simulink model "foureightbits_thirtytwobit"  (Simulink 7.8)
settings: Solver=FixedStepDiscrete  StartTime=0.0  StopTime=10.0  RelTol=1e-3
settings Model: Creator=Embed_Sys_course  LastModifiedBy=Embed_Sys_course
settings DataIOCC: ExternalInput=off  InitialState=off  SaveOutput=off  SignalLogging=off  SaveTime=off
settings OptimizationCC: InlineParams=on  OptimizeModelRefInitCode=on  LifeSpan=1
settings DebuggingCC: InheritedTsInSrcMsg=none  SingleTaskRateTransMsg=error  UnderSpecifiedDataTypeMsg=error  UnnecessaryDatatypeConvMsg=warning  UnconnectedInputMsg=error  UnconnectedOutputMsg=error  UnconnectedLineMsg=error  UnknownTsInhSupMsg=error
settings HardwareCC: ProdLargestAtomicInteger=Long  ProdLargestAtomicFloat=Double  ProdIntDivRoundTo=Zero  ProdEndianess=BigEndian  ProdHWDeviceType=Motorola PowerPC
settings RTWCC: SystemTargetFile=ert.tlc  TemplateMakefile=ert_default_tmf  Description=Embedded Coder  GenerateReport=on  ProcessScript=ert_make_rtw_hook  IncludeHyperlinkInReport=on  LaunchReport=on  GenerateTraceInfo=on  GenerateTraceReport=on  GenerateTraceReportSl=on  GenerateTraceReportSf=on  GenerateTraceReportEml=on  GenerateCodeMetricsReport=on
settings CodeAppCC: IgnoreCustomStorageClasses=off
settings ERTTargetCC: MultiwordLength=2048  GenerateSampleERTMain=on  InlinedParameterPlacement=NonHierarchical  ERTCustomFileTemplate=example_file_process.tlc  ConvertIfToSwitch=off  SuppressUnreachableDefaultCases=off

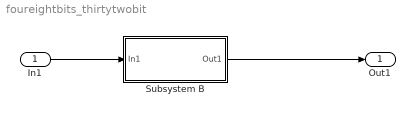
== system foureightbits_thirtytwobit ==
  In1 : Inport  OutDataTypeStr=uint8  PortDimensions=4
  Subsystem B : Subsystem
  Out1 : Outport  OutDataTypeStr=uint32
  wires:
  In1/1 -> Subsystem B/1(In1)
  Subsystem B/1(Out1) -> Out1/1

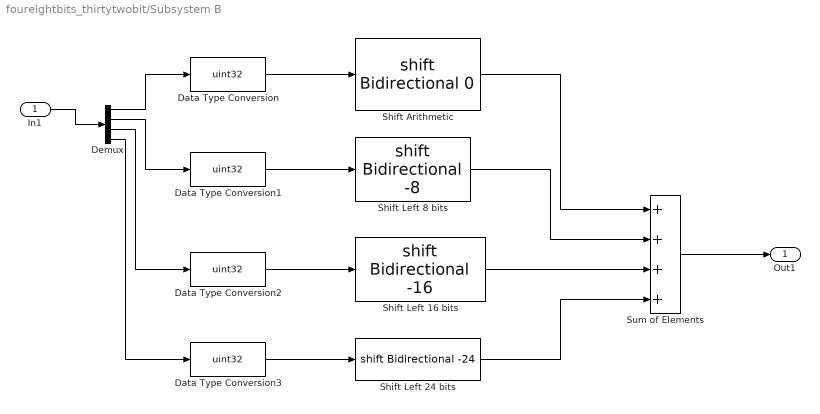
== system foureightbits_thirtytwobit/Subsystem B ==
  In1 : Inport
  Data Type Conversion{,1..3} (4 alike) : DataTypeConversion  OutDataTypeStr=uint32
  Demux : Demux
  Shift Arithmetic : ArithShift
  Shift Left 16 bits : ArithShift  BitShiftNumber=-16
  Shift Left 24 bits : ArithShift  BitShiftNumber=-24
  Shift Left 8 bits : ArithShift  BitShiftNumber=-8
  Sum of Elements : Sum  Inputs=++++
  Out1 : Outport
  wires:
  In1/1 -> Demux/1
  Sum of Elements/1 -> Out1/1
  Data Type Conversion/1 -> Shift Arithmetic/1
  Data Type Conversion1/1 -> Shift Left 8 bits/1
  Data Type Conversion2/1 -> Shift Left 16 bits/1
  Data Type Conversion3/1 -> Shift Left 24 bits/1
  Demux/1 -> Data Type Conversion/1
  Demux/2 -> Data Type Conversion1/1
  Demux/3 -> Data Type Conversion2/1
  Demux/4 -> Data Type Conversion3/1
  Shift Arithmetic/1 -> Sum of Elements/1
  Shift Left 8 bits/1 -> Sum of Elements/2
  Shift Left 16 bits/1 -> Sum of Elements/3
  Shift Left 24 bits/1 -> Sum of Elements/4
